simulink subsystem "diffrential_model_of_slab (1)"  (R2024a)
settings: Solver=VariableStepAuto  StartTime=0.0  StopTime=10.0  RelTol=1e-3

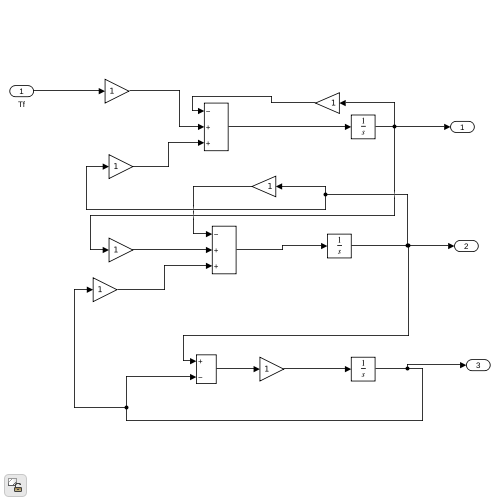
[thumbnail: Simulink's stored preview of the top-level diagram]
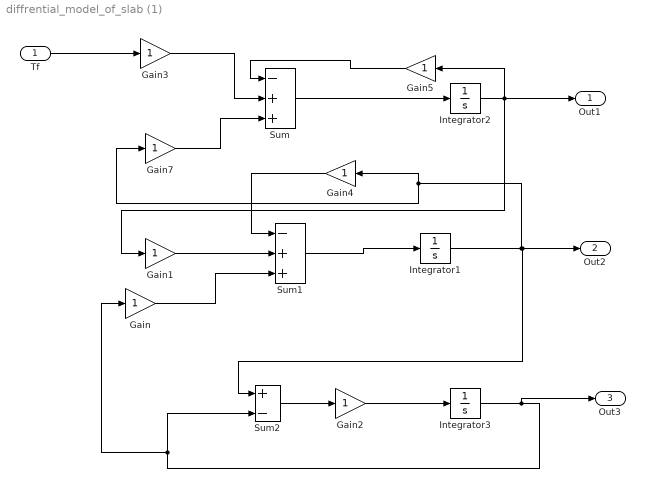
== system diffrential_model_of_slab (1) ==
  Tf : Inport
  Gain{,1..5,7} (7 alike) : Gain
  Integrator1 : Integrator
  Integrator2 : Integrator
  Integrator3 : Integrator
  Sum : Sum  Inputs=-|+|+
  Sum1 : Sum  Inputs=-|+|+
  Sum2 : Sum  Inputs=+|-
  Out1 : Outport
  Out2 : Outport  Port=2
  Out3 : Outport  Port=3
  wires:
  Tf/1 -> Gain3/1
  Integrator3/1 -> Gain/1, Sum2/2, Out3/1
  Gain7/1 -> Sum/3
  Gain2/1 -> Integrator3/1
  Gain3/1 -> Sum/2
  Integrator1/1 -> Gain4/1, Gain7/1, Sum2/1, Out2/1
  Sum/1 -> Integrator2/1
  Sum2/1 -> Gain2/1
  Integrator2/1 -> Gain5/1, Gain1/1, Out1/1
  Gain4/1 -> Sum1/1
  Sum1/1 -> Integrator1/1
  Gain1/1 -> Sum1/2
  Gain5/1 -> Sum/1
  Gain/1 -> Sum1/3
